simulink model "task4"  (R2023a)
settings: Solver=VariableStepAuto  StartTime=0.0  StopTime=20.0  RelTol=1e-8
settings Model: Creator=vasil  LastModifiedBy=vasil

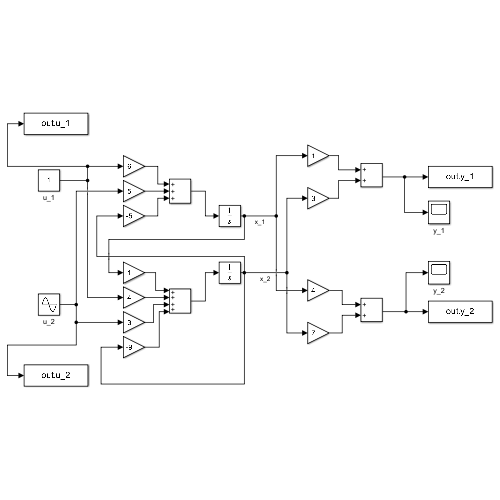
[thumbnail: Simulink's stored preview of the top-level diagram]
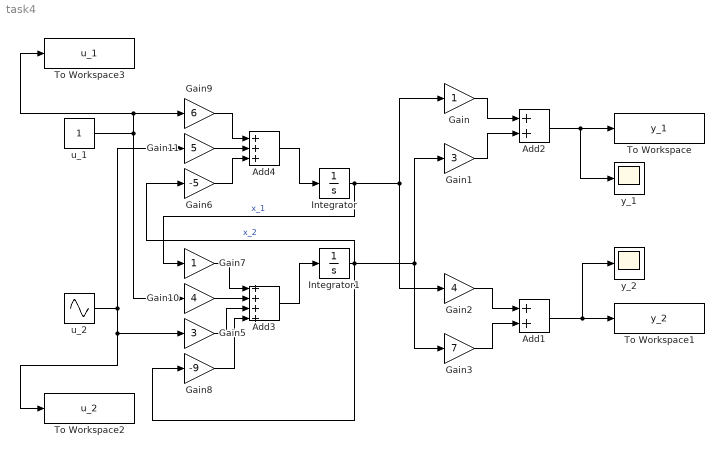
== system task4 ==
  Add1 : Sum
  Add2 : Sum
  Add3 : Sum  Inputs=++++
  Add4 : Sum  Inputs=+++
  Gain : Gain
  Gain1 : Gain  Gain=3
  Gain10 : Gain  Gain=4
  Gain11 : Gain  Gain=5
  Gain2 : Gain  Gain=4
  Gain3 : Gain  Gain=7
  Gain5 : Gain  Gain=3
  Gain6 : Gain  Gain=-5
  Gain7 : Gain
  Gain8 : Gain  Gain=-9
  Gain9 : Gain  Gain=6
  Integrator : Integrator
  Integrator1 : Integrator
  To Workspace : ToWorkspace  VariableName=y_1  SaveFormat=Timeseries  SampleTime=-1
  To Workspace1 : ToWorkspace  VariableName=y_2  SaveFormat=Timeseries  SampleTime=-1
  To Workspace2 : ToWorkspace  VariableName=u_2  SaveFormat=Timeseries  SampleTime=-1
  To Workspace3 : ToWorkspace  VariableName=u_1  SaveFormat=Timeseries  SampleTime=-1
  u_1 : Constant
  u_2 : Sin  Amplitude=2  SampleTime=0
  y_1 : Scope
  y_2 : Scope
  wires:
  Add2/1 -> y_1/1, To Workspace/1
  u_2/1 -> Gain11/1, Gain5/1, To Workspace2/1
  u_1/1 -> Gain9/1, To Workspace3/1, Gain10/1
  Add1/1 -> y_2/1, To Workspace1/1
  Gain1/1 -> Add2/2
  Gain/1 -> Add2/1
  Gain2/1 -> Add1/1
  Gain3/1 -> Add1/2
  Integrator1/1 -> Gain1/1, Gain3/1, Gain8/1, Gain6/1  "x_2"
  Integrator/1 -> Gain7/1, Gain/1, Gain2/1  "x_1"
  Add3/1 -> Integrator1/1
  Add4/1 -> Integrator/1
  Gain7/1 -> Add3/1
  Gain8/1 -> Add3/4
  Gain5/1 -> Add3/3
  Gain10/1 -> Add3/2
  Gain9/1 -> Add4/1
  Gain6/1 -> Add4/3
  Gain11/1 -> Add4/2
